simulink model "simple"  (R2017a)
settings: Solver=FixedStepDiscrete  StartTime=0.0  StopTime=10  RelTol=1e-3
settings Model: DataTypeOverride=Off  Creator=mini  LastModifiedBy=mini
settings DataIOCC: SaveOutput=off  SaveTime=off
settings OptimizationCC: BlockReduction=off  ConditionallyExecuteInputs=off  DefaultParameterBehavior=Inlined
settings DebuggingCC: AlgebraicLoopMsg=error  SingleTaskRateTransMsg=error  StrictBusMsg=ErrorOnBusTreatedAsVector
settings HardwareCC: ProdBitPerPointer=32  ProdBitPerSizeT=32  ProdBitPerPtrDiffT=32  ProdLargestAtomicFloat=None  ProdIntDivRoundTo=Undefined  ProdEndianess=Unspecified  ProdWordSize=32  ProdHWDeviceType=ASIC/FPGA->ASIC/FPGA  ProdEqTarget=off
settings GRTTargetCC: TargetLangStandard=C89/C90 (ANSI)

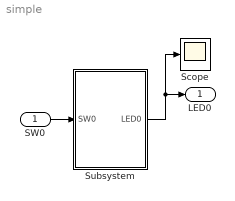
== system simple ==
  SW0 : Inport  OutDataTypeStr=boolean
  Scope : Scope
  Subsystem : Subsystem  TreatAsAtomicUnit=on
  LED0 : Outport
  wires:
  SW0/1 -> Subsystem/1(SW0)
  Subsystem/1(LED0) -> Scope/1, LED0/1

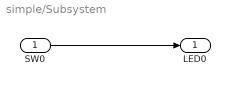
== system simple/Subsystem ==
  SW0 : Inport  OutDataTypeStr=boolean
  LED0 : Outport  SampleTime=10
  wires:
  SW0/1 -> LED0/1
